simulink subsystem "v2021_10_27_Gear"  (R2020b)
settings: Solver=VariableStepAuto  StartTime=0.0  StopTime=10.0  RelTol=1e-3
values from neighbouring files (symbols this model uses):
  coeffAttritoStatico = 0.7    [v2021_10_27_avvioSITL.m]
  costantiMagicFormula = [ 10 1.3 1 0.95 ]    [v2021_10_27_avvioSITL.m]
  limitAinf = -500    [v2021_10_27_avvioSITL.m]
  limitAup = 500    [v2021_10_27_avvioSITL.m]
  limitPinf = -500    [v2021_10_27_avvioSITL.m]
  limitPup = 500    [v2021_10_27_avvioSITL.m]
  massaRuotaAnteriore = m    [v2021_10_27_avvioSITL.m]
  massaRuotePosteriori = m    [v2021_10_27_avvioSITL.m]
  Zpista = 0    [v2021_10_27_avvioSITL.m]
libraries: sharedutil x12, vrlib x9, simulink x1
(part 1 of 2)
settings Model: Creator=Simone  LastModifiedBy=emanueledalessio

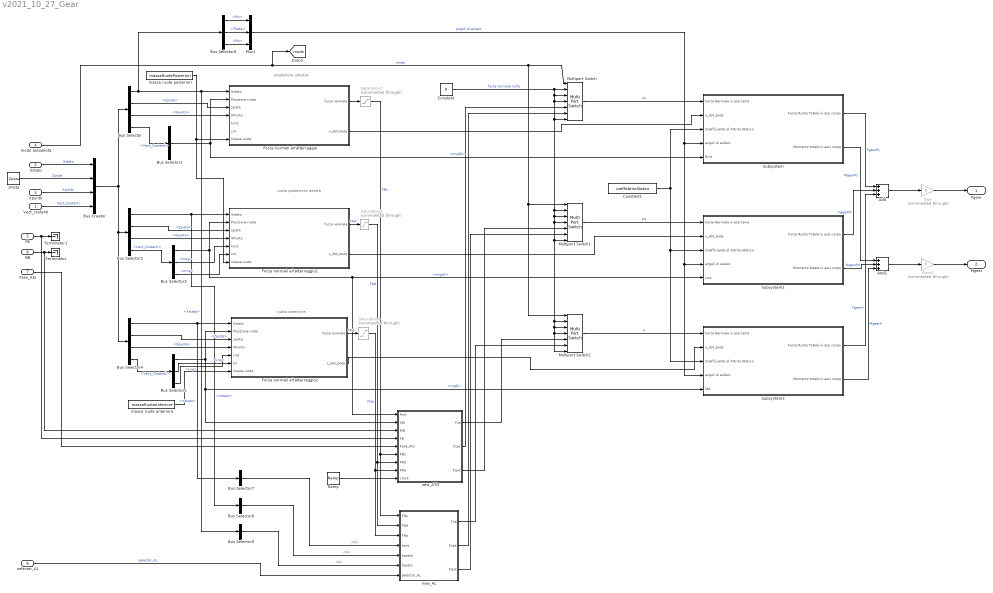
== system v2021_10_27_Gear ==
  note: ruota anteriore
  note: ruota posteriore destra
  note: posteriore sinistra
  Vect_costanti : Inport
  Xstato : Inport  Port=2
  Xpunto : Inport  Port=3
  modo autopilota : Inport  Port=4
  FB : Inport  Port=5
  MB : Inport  Port=6
  Fase_Ato : Inport  Port=7
  selector_AL : Inport  Port=8
  Add : Sum  Inputs=+++
  Add1 : Sum  Inputs=+++
  Bus Creator : BusCreator  Inputs=4
  Bus Selector : BusSelector  OutputSignals=Xstato,Zpista,Xpunto,Vect_Costanti
  Bus Selector1 : BusSelector  OutputSignals=Vett_caratteristici.rmglG
  Bus Selector2 : BusSelector  OutputSignals=Xstato,Zpista,Xpunto,Vect_Costanti
  Bus Selector3 : BusSelector  OutputSignals=Vett_caratteristici.rmgrG,gear.kmg,gear.cmg
  Bus Selector4 : BusSelector  OutputSignals=Xstato,Zpista,Xpunto,Vect_Costanti
  Bus Selector5 : BusSelector  OutputSignals=Vett_caratteristici.rngG,gear.kng,gear.cng
  Bus Selector6 : BusSelector  OutputSignals=PhiThetaPsi.Phi,PhiThetaPsi.Theta,PhiThetaPsi.Psi
  Bus Selector7 : BusSelector  OutputSignals=xyz.h
  Bus Selector8 : BusSelector  OutputSignals=xyz.h
  Bus Selector9 : BusSelector  OutputSignals=xyz.h
  Constant : Constant  Value=0
  Constant1 : Constant  Value=coeffAttritoStatico
  Forze normali all'atterraggio : Subsystem
  Forze normali all'atterraggio1 : Subsystem
  Forze normali all'atterraggio2 : Subsystem
  Gain : Gain  Commented=through  Gain=0
  Gain1 : Gain  Commented=through  Gain=0
  Multiport Switch : MultiPortSwitch  DataPortOrder=Specify indices  DataPortIndices={0,1,2,3,4,5}
  Multiport Switch1 : MultiPortSwitch  DataPortOrder=Specify indices  DataPortIndices={0,1,2,3,4,5}
  Multiport Switch2 : MultiPortSwitch  DataPortOrder=Specify indices  DataPortIndices={0,1,2,3,4,5}
  Mux1 : Mux  Inputs=3
  Ramp : simulink/Sources/Ramp  slope=1  start=0  InitialOutput=0
  Saturation2 : Saturate  Commented=through  UpperLimit=600  LowerLimit=-600
  Saturation3 : Saturate  Commented=through  UpperLimit=600  LowerLimit=-600
  Saturation4 : Saturate  Commented=through  UpperLimit=950  LowerLimit=-950
  Subsystem : Subsystem
  Subsystem1 : Subsystem
  Subsystem2 : Subsystem
  Terminator : Terminator
  Terminator1 : Terminator
  massa ruota anteriore : Constant  Value=massaRuotaAnteriore
  massa ruote posteriori : Constant  Value=massaRuotePosteriori
  new_AL : MATLAB Function  TreatAsAtomicUnit=on
  new_ATO : MATLAB Function  TreatAsAtomicUnit=on
  zPista : Constant  Value=Zpista
  Fgear : Outport  VectorParamsAs1DForOutWhenUnconnected=off
  Mgear : Outport  Port=2  VectorParamsAs1DForOutWhenUnconnected=off
  tag scope: modo=global
  wires:
  Constant1/1 -> Subsystem/3(Coefficiente di Attrito Statico), Subsystem1/3(Coefficiente di Attrito Statico), Subsystem2/3(Coefficiente di Attrito Statico)
  Bus Selector1/1 -> Subsystem/5(Rmt), Forze normali all'atterraggio/2(Posizione ruota)  "<rmglG>"
  Subsystem/2(Momento totale in assi corpo) -> Add1/1  "MgearPs"
  massa ruota anteriore/1 -> Forze normali all'atterraggio2/7(massa ruota)
  Forze normali all'atterraggio/1(forza normale) -> Saturation2/1
  Forze normali all'atterraggio2/2(x_dot_body) -> Subsystem2/2(x_dot_body)
  Forze normali all'atterraggio1/1(forza normale) -> Saturation3/1  "FNd"
  modo autopilota/1 -> Multiport Switch/1, Multiport Switch1/1, Multiport Switch2/1, [modo]  "modo"
  Add/1 -> Gain/1
  Add1/1 -> Gain1/1
  Constant/1 -> Multiport Switch/2, Multiport Switch/3, Multiport Switch1/2, Multiport Switch1/3, Multiport Switch2/2, Multiport Switch2/3, Multiport Switch2/7, Multiport Switch2/4, Multiport Switch1/7, Multiport Switch1/4, Multiport Switch/7, Multiport Switch/4  "forza normale nulla"
  Bus Selector6/2 -> Mux1/2  "<Theta>"
  Bus Selector4/4 -> Bus Selector5/1  "<Vect_Costanti>"
  Subsystem2/2(Momento totale in assi corpo) -> Add1/3  "MgearA"
  ? -> Forze normali all'atterraggio/5(kmd)  "<kmg>"
  Bus Selector5/3 -> Forze normali all'atterraggio2/5(cnd)  "<cng>"
  Bus Selector6/3 -> Mux1/3  "<Psi>"
  Fase_Ato/1 -> new_ATO/5(Fase_Ato)
  Bus Creator/1 -> Bus Selector/1, Bus Selector2/1, Bus Selector4/1
  Bus Selector2/1 -> Forze normali all'atterraggio1/1(Xstato), Bus Selector8/1  "<Xstato>"
  Xpunto/1 -> Bus Creator/3  "Xpunto"
  Bus Selector4/1 -> Forze normali all'atterraggio2/1(Xstato), Bus Selector7/1  "<Xstato>"
  Bus Selector2/4 -> Bus Selector3/1  "<Vect_Costanti>"
  Forze normali all'atterraggio1/2(x_dot_body) -> Subsystem1/2(x_dot_body)
  Xstato/1 -> Bus Creator/1  "Xstato"
  Multiport Switch1/1 -> Subsystem1/1(Forza Normale in assi terra)  "Pd"
  Subsystem1/2(Momento totale in assi corpo) -> Add1/2  "MgearPd"
  Bus Selector/4 -> Bus Selector1/1  "<Vect_Costanti>"
  Multiport Switch/1 -> Subsystem/1(Forza Normale in assi terra)  "Ps"
  Subsystem1/1(Forza Ruota Totale in assi corpo) -> Add/2  "FgearPd"
  Forze normali all'atterraggio/2(x_dot_body) -> Subsystem/2(x_dot_body)
  Subsystem2/1(Forza Ruota Totale in assi corpo) -> Add/3  "FgearA"
  zPista/1 -> Bus Creator/2  "Zpista"
  Bus Selector/1 -> Forze normali all'atterraggio/1(Xstato), Bus Selector9/1, Bus Selector6/1  "<Xstato>"
  massa ruote posteriori/1 -> Forze normali all'atterraggio/7(massa ruota), Forze normali all'atterraggio1/7(massa ruota)
  Bus Selector2/3 -> Forze normali all'atterraggio1/4(XPunto)  "<Xpunto>"
  Bus Selector6/1 -> Mux1/1  "<Phi>"
  ? -> Forze normali all'atterraggio/6(cm)  "<cmg>"
  Bus Selector/3 -> Forze normali all'atterraggio/4(XPunto)  "<Xpunto>"
  Bus Selector5/2 -> Forze normali all'atterraggio2/6(kn)  "<kng>"
  Bus Selector2/2 -> Forze normali all'atterraggio1/3(zpista)  "<Zpista>"
  Bus Selector/2 -> Forze normali all'atterraggio/3(zpista)  "<Zpista>"
  Bus Selector3/1 -> Forze normali all'atterraggio1/2(Posizione ruota), Subsystem1/5(Lmt), new_ATO/1(Rmt)  "<rmgrG>"
  Vect_costanti/1 -> Bus Creator/4  "Vect_Costanti"
  Forze normali all'atterraggio2/1(forza normale) -> Saturation4/1  "FNa"
  Multiport Switch2/1 -> Subsystem2/1(Forza Normale in assi terra)  "A"
  Bus Selector5/1 -> Forze normali all'atterraggio2/2(Posizione ruota), new_ATO/2(Sbt), Subsystem2/5(Sbt)  "<rngG>"
  Subsystem/1(Forza Ruota Totale in assi corpo) -> Add/1  "FgearPs"
  Mux1/1 -> Subsystem/4(angoli di eulero), Subsystem1/4(angoli di eulero), Subsystem2/4(angoli di eulero)  "angoli di eulero"
  Bus Selector4/3 -> Forze normali all'atterraggio2/4(XPunto)  "<Xpunto>"
  Bus Selector4/2 -> Forze normali all'atterraggio2/3(zpista)  "<Zpista>"
  new_ATO/1(Fza) -> Multiport Switch2/5
  Bus Selector3/3 -> Forze normali all'atterraggio1/6(cm)  "<cmg>"
  Bus Selector3/2 -> Forze normali all'atterraggio1/5(kmd)  "<kmg>"
  FB/1 -> Terminator1/1, new_ATO/4(FB)
  Saturation2/1 -> new_AL/1(FNs), new_ATO/6(FNs)  "FNs"
  Saturation3/1 -> new_AL/2(FNd), new_ATO/7(FNd)  "FNd"
  Saturation4/1 -> new_ATO/8(FNa), new_AL/3(FNa)  "FNa"
  new_ATO/2(Fzps) -> Multiport Switch/5
  new_ATO/3(Fzpd) -> Multiport Switch1/5
  Ramp/1 -> new_ATO/9(clock)
  MB/1 -> Terminator/1, new_ATO/3(MB)
  Gain1/1 -> Mgear/1
  Gain/1 -> Fgear/1
  new_AL/1(Fza) -> Multiport Switch2/6
  new_AL/3(Fzpd) -> Multiport Switch1/6
  new_AL/2(Fzps) -> Multiport Switch/6
  Bus Selector7/1 -> new_AL/4(hant)  "<h>"
  Bus Selector8/1 -> new_AL/5(hpostd)  "<h>"
  Bus Selector9/1 -> new_AL/6(hposts)  "<h>"
  selector_AL/1 -> new_AL/7(selector_AL)  "selector_AL"

== system v2021_10_27_Gear/Forze normali all'atterraggio ==
  note: ruota posteriore sinistra
  note: CINEMATICA RUOTE
  Xstato : Inport
  Posizione ruota : Inport  Port=2
  zpista : Inport  Port=3
  XPunto : Inport  Port=4
  kmd : Inport  Port=5
  cm : Inport  Port=6
  massa ruota : Inport  Port=7
  Demux : Demux  Outputs=3
  Demux4 : Demux  Outputs=3
  Subsystem5 : Subsystem
  Terminator{,1..3} (4 alike) : Terminator
  cinematica : Subsystem
  forza normale : Outport
  x_dot_body : Outport  Port=2
  wires:
  cm/1 -> Subsystem5/5(km)
  kmd/1 -> Subsystem5/4(cmd)
  massa ruota/1 -> Subsystem5/6(massa ruota)
  Subsystem5/1(forza normale) -> forza normale/1
  XPunto/1 -> cinematica/4(XPunto)
  zpista/1 -> cinematica/3(Zpista)
  Posizione ruota/1 -> cinematica/2(Posisione Ruota)
  Xstato/1 -> cinematica/1(Xstato)
  cinematica/3(accelerazione ruota rispetto al terreno) -> Demux/1  "x_dot_dot"
  cinematica/1(distanza verticale ruota pista) -> Subsystem5/1(h)  "hps"
  cinematica/2(velocità ruota rispetto al terreno) -> Demux4/1  "x_dot"
  Demux/1 -> Terminator1/1  "x_dot_dot"
  Demux4/2 -> Terminator2/1  "y_dot"
  Demux4/1 -> Terminator3/1  "x_dot"
  Demux4/3 -> Subsystem5/2(h_dot)  "h_dot"
  Demux/3 -> Subsystem5/3(h_dot_dot)  "h_dot dot"
  cinematica/4(velocità ruota rispetto al terreno in assi corpo) -> x_dot_body/1  "x_dot_body"
  Demux/2 -> Terminator/1  "y_dot_dot"

== system v2021_10_27_Gear/Forze normali all'atterraggio1 ==
  note: ruota posteriore sinistra
  note: CINEMATICA RUOTE
  Xstato : Inport
  Posizione ruota : Inport  Port=2
  zpista : Inport  Port=3
  XPunto : Inport  Port=4
  kmd : Inport  Port=5
  cm : Inport  Port=6
  massa ruota : Inport  Port=7
  Demux : Demux  Outputs=3
  Demux4 : Demux  Outputs=3
  Subsystem5 : Subsystem
  Terminator{,1..3} (4 alike) : Terminator
  cinematica : Subsystem
  forza normale : Outport
  x_dot_body : Outport  Port=2
  wires:
  cm/1 -> Subsystem5/5(km)
  kmd/1 -> Subsystem5/4(cmd)
  massa ruota/1 -> Subsystem5/6(massa ruota)
  Subsystem5/1(forza normale) -> forza normale/1
  XPunto/1 -> cinematica/4(XPunto)
  zpista/1 -> cinematica/3(Zpista)
  Posizione ruota/1 -> cinematica/2(Posisione Ruota)
  Xstato/1 -> cinematica/1(Xstato)
  cinematica/3(accelerazione ruota rispetto al terreno) -> Demux/1  "x_dot_dot"
  cinematica/1(distanza verticale ruota pista) -> Subsystem5/1(h)  "hpd"
  cinematica/2(velocità ruota rispetto al terreno) -> Demux4/1  "x_dot"
  Demux/1 -> Terminator1/1  "x_dot_dot"
  Demux4/2 -> Terminator2/1  "y_dot"
  Demux4/1 -> Terminator3/1  "x_dot"
  Demux4/3 -> Subsystem5/2(h_dot)  "h_dot"
  Demux/3 -> Subsystem5/3(h_dot_dot)  "h_dot dot"
  cinematica/4(velocità ruota rispetto al terreno in assi corpo) -> x_dot_body/1  "x_dot_body"
  Demux/2 -> Terminator/1  "y_dot_dot"

== system v2021_10_27_Gear/Forze normali all'atterraggio2 ==
  note: ruota posteriore sinistra
  note: CINEMATICA RUOTE
  Xstato : Inport
  Posizione ruota : Inport  Port=2
  zpista : Inport  Port=3
  XPunto : Inport  Port=4
  cnd : Inport  Port=5
  kn : Inport  Port=6
  massa ruota : Inport  Port=7
  Demux : Demux  Outputs=3
  Demux4 : Demux  Outputs=3
  Subsystem5 : Subsystem
  Terminator{,1..3} (4 alike) : Terminator
  cinematica : Subsystem
  forza normale : Outport
  x_dot_body : Outport  Port=2
  wires:
  kn/1 -> Subsystem5/5(kn)
  cnd/1 -> Subsystem5/4(cnd)
  massa ruota/1 -> Subsystem5/6(massa ruota)
  Subsystem5/1(forza normale) -> forza normale/1
  XPunto/1 -> cinematica/4(XPunto)
  zpista/1 -> cinematica/3(Zpista)
  Posizione ruota/1 -> cinematica/2(Posisione Ruota)
  Xstato/1 -> cinematica/1(Xstato)
  cinematica/3(accelerazione ruota rispetto al terreno) -> Demux/1  "x_dot_dot"
  cinematica/1(distanza verticale ruota pista) -> Subsystem5/1(h)  "ha"
  cinematica/2(velocità ruota rispetto al terreno) -> Demux4/1  "x_dot"
  Demux/1 -> Terminator1/1  "x_dot_dot"
  Demux4/2 -> Terminator2/1  "y_dot"
  Demux4/1 -> Terminator3/1  "x_dot"
  Demux4/3 -> Subsystem5/2(h_dot)  "h_dot"
  Demux/3 -> Subsystem5/3(h_dot_dot)  "h_dot dot"
  cinematica/4(velocità ruota rispetto al terreno in assi corpo) -> x_dot_body/1  "x_dot_body"
  Demux/2 -> Terminator/1  "y_dot_dot"

== system v2021_10_27_Gear/Subsystem ==
  note: di solito: B = 10
      | 		C = 1.3
      | 		D = 1
      | 		E = 0.95
  Forza Normale in assi terra : Inport
  x_dot_body : Inport  Port=2
  Coefficiente di Attrito Statico : Inport  Port=3
  angoli di eulero : Inport  Port=4
  Rmt : Inport  Port=5
  Atan : Trigonometry  Operator=atan
  Constant : Constant  Value=0
  Cross Product : vrlib/Utilities/Cross Product
  Demux : Demux  Outputs=3
  Demux1 : Demux
  Demux2 : Demux  Outputs=3
  Divide : Product  Inputs=*/
  Gain : Gain  Commented=through  Gain=-1
  Gain1 : Gain  Gain=-1
  Gain3 : Gain  Gain=-1
  Gain4 : Gain  Commented=through  Gain=0
  MATLAB Function1 : MATLAB Function  TreatAsAtomicUnit=on
  MATLAB Function3 : MATLAB Function  TreatAsAtomicUnit=on
  Mux : Mux  Inputs=3
  Mux1 : Mux  Inputs=3
  Product : Product
  Saturation : Saturate  UpperLimit=0  LowerLimit=-1000000
  Subsystem : Subsystem
  Terminator : Terminator
  Terminator1 : Terminator
  Terminator2 : Terminator
  Vettore Coefficienti Magic Formula : Constant  Value=costantiMagicFormula  VectorParams1D=off
  Forza Ruota Totale in assi corpo : Outport
  Momento totale in assi corpo : Outport  Port=2
  wires:
  Gain1/1 -> Mux/1
  Gain4/1 -> Mux/3
  Gain3/1 -> Mux1/3
  Forza Normale in assi terra/1 -> Product/1, Gain3/1
  Gain/1 -> Saturation/1
  Saturation/1 -> MATLAB Function1/6(Fa)
  MATLAB Function3/1(forza_normale) -> Gain/1
  Mux1/1 -> Subsystem/2(Input1)
  Demux2/3 -> Gain4/1
  Demux2/2 -> Terminator2/1
  Demux2/1 -> Terminator1/1
  Subsystem/1(Output) -> Demux2/1  "forza normale in assi corpo"
  Product/1 -> MATLAB Function3/1(forzanormale)  "Fa max"
  Demux1/4 -> MATLAB Function1/4(E)  "E"
  Demux1/3 -> MATLAB Function1/3(D)  "D"
  Demux1/2 -> MATLAB Function1/2(C)  "C"
  Demux1/1 -> MATLAB Function1/1(B)  "B"
  Vettore Coefficienti Magic Formula/1 -> Demux1/1
  Cross Product/1 -> Momento totale in assi corpo/1
  Rmt/1 -> Cross Product/1
  angoli di eulero/1 -> Subsystem/1(Input)
  Constant/1 -> Mux1/1, Mux1/2
  Mux/1 -> Forza Ruota Totale in assi corpo/1, Cross Product/2
  MATLAB Function1/2(Fy) -> Mux/2  "Fy"
  MATLAB Function1/1(Fx) -> Gain1/1  "Fx"
  Demux/1 -> Divide/2
  Atan/1 -> MATLAB Function1/5(beta)  "Angolo di Deriva beta"
  Divide/1 -> Atan/1
  Demux/2 -> Divide/1
  Demux/3 -> Terminator/1
  Coefficiente di Attrito Statico/1 -> Product/2
  x_dot_body/1 -> Demux/1  "vettore velocità ruota in assi corpo"

== system v2021_10_27_Gear/Subsystem1 ==
  note: di solito: B = 10
      | 		C = 1.3
      | 		D = 1
      | 		E = 0.95
  Forza Normale in assi terra : Inport
  x_dot_body : Inport  Port=2
  Coefficiente di Attrito Statico : Inport  Port=3
  angoli di eulero : Inport  Port=4
  Lmt : Inport  Port=5
  Atan : Trigonometry  Operator=atan
  Constant : Constant  Value=0
  Cross Product : vrlib/Utilities/Cross Product
  Demux : Demux  Outputs=3
  Demux1 : Demux
  Demux2 : Demux  Outputs=3
  Divide : Product  Inputs=*/
  Gain : Gain  Commented=through  Gain=-1
  Gain1 : Gain  Gain=-1
  Gain3 : Gain  Gain=-1
  Gain4 : Gain  Commented=through  Gain=0
  MATLAB Function1 : MATLAB Function  TreatAsAtomicUnit=on
  MATLAB Function3 : MATLAB Function  TreatAsAtomicUnit=on
  Mux : Mux  Inputs=3
  Mux1 : Mux  Inputs=3
  Product : Product
  Saturation : Saturate  UpperLimit=0  LowerLimit=-1000000
  Subsystem : Subsystem
  Terminator : Terminator
  Terminator1 : Terminator
  Terminator2 : Terminator
  Vettore Coefficienti Magic Formula1 : Constant  Value=costantiMagicFormula  VectorParams1D=off
  Forza Ruota Totale in assi corpo : Outport
  Momento totale in assi corpo : Outport  Port=2
  wires:
  Gain4/1 -> Mux/3
  Gain1/1 -> Mux1/3
  Gain3/1 -> Mux/1
  MATLAB Function3/1(forza_normale) -> Gain/1
  Gain/1 -> Saturation/1
  Saturation/1 -> MATLAB Function1/6(Fa)
  Demux2/3 -> Gain4/1
  Subsystem/1(Output) -> Demux2/1  "forza normale in assi corpo"
  Demux2/2 -> Terminator2/1
  Demux2/1 -> Terminator1/1
  Forza Normale in assi terra/1 -> Gain1/1, Product/1
  Product/1 -> MATLAB Function3/1(forzanormale)  "Fa max"
  Demux1/4 -> MATLAB Function1/4(E)  "E"
  Demux1/3 -> MATLAB Function1/3(D)  "D"
  Demux1/2 -> MATLAB Function1/2(C)  "C"
  Demux1/1 -> MATLAB Function1/1(B)  "B"
  Vettore Coefficienti Magic Formula1/1 -> Demux1/1
  Cross Product/1 -> Momento totale in assi corpo/1
  Lmt/1 -> Cross Product/1
  Mux1/1 -> Subsystem/2(Input1)
  angoli di eulero/1 -> Subsystem/1(Input)
  Constant/1 -> Mux1/1, Mux1/2
  Mux/1 -> Forza Ruota Totale in assi corpo/1, Cross Product/2
  MATLAB Function1/2(Fy) -> Mux/2  "Fy"
  MATLAB Function1/1(Fx) -> Gain3/1  "Fx"
  Demux/1 -> Divide/2
  Atan/1 -> MATLAB Function1/5(beta)  "Angolo di Deriva beta"
  Divide/1 -> Atan/1
  Demux/2 -> Divide/1
  Demux/3 -> Terminator/1
  Coefficiente di Attrito Statico/1 -> Product/2
  x_dot_body/1 -> Demux/1  "vettore velocità ruota in assi corpo"

== system v2021_10_27_Gear/Subsystem2 ==
  note: di solito: B = 10
      | 		C = 1.3
      | 		D = 1
      | 		E = 0.95
  Forza Normale in assi terra : Inport
  x_dot_body : Inport  Port=2
  Coefficiente di Attrito Statico : Inport  Port=3
  angoli di eulero : Inport  Port=4
  Sbt : Inport  Port=5
  Atan : Trigonometry  Operator=atan
  Constant : Constant  Value=0
  Cross Product : vrlib/Utilities/Cross Product
  Demux : Demux  Outputs=3
  Demux1 : Demux
  Demux2 : Demux  Outputs=3
  Divide : Product  Inputs=*/
  Gain : Gain  Commented=through  Gain=-1
  Gain2 : Gain  Gain=-1
  Gain3 : Gain  Gain=-1
  Gain4 : Gain  Commented=through  Gain=0
  MATLAB Function1 : MATLAB Function  TreatAsAtomicUnit=on
  MATLAB Function3 : MATLAB Function  TreatAsAtomicUnit=on
  Mux : Mux  Inputs=3
  Mux1 : Mux  Inputs=3
  Product : Product
  Saturation : Saturate  UpperLimit=0  LowerLimit=-1000000
  Subsystem : Subsystem
  Terminator : Terminator
  Terminator1 : Terminator
  Terminator2 : Terminator
  Vettore Coefficienti Magic Formula : Constant  Value=costantiMagicFormula  VectorParams1D=off
  Forza Ruota Totale in assi corpo : Outport
  Momento totale in assi corpo : Outport  Port=2
  wires:
  Gain4/1 -> Mux/3
  Gain3/1 -> Mux1/3
  Gain2/1 -> Mux/1
  Gain/1 -> Saturation/1
  Saturation/1 -> MATLAB Function1/6(Fa)
  MATLAB Function3/1(forza_normale) -> Gain/1
  Mux1/1 -> Subsystem/2(Input1)
  Demux2/3 -> Gain4/1
  Subsystem/1(Output) -> Demux2/1  "forza normale in assi corpo"
  Demux2/2 -> Terminator2/1
  Demux2/1 -> Terminator1/1
  Forza Normale in assi terra/1 -> Gain3/1, Product/1
  Product/1 -> MATLAB Function3/1(forzanormale)  "Fa max"
  Demux1/4 -> MATLAB Function1/4(E)  "E"
  Demux1/3 -> MATLAB Function1/3(D)  "D"
  Demux1/2 -> MATLAB Function1/2(C)  "C"
  Demux1/1 -> MATLAB Function1/1(B)  "B"
  Vettore Coefficienti Magic Formula/1 -> Demux1/1
  Cross Product/1 -> Momento totale in assi corpo/1
  Sbt/1 -> Cross Product/1
  angoli di eulero/1 -> Subsystem/1(Input)
  Constant/1 -> Mux1/1, Mux1/2
  Mux/1 -> Forza Ruota Totale in assi corpo/1, Cross Product/2
  MATLAB Function1/2(Fy) -> Mux/2  "Fy"
  MATLAB Function1/1(Fx) -> Gain2/1  "Fx"
  Demux/1 -> Divide/2
  Atan/1 -> MATLAB Function1/5(beta)  "Angolo di Deriva beta"
  Divide/1 -> Atan/1
  Demux/2 -> Divide/1
  Demux/3 -> Terminator/1
  Coefficiente di Attrito Statico/1 -> Product/2
  x_dot_body/1 -> Demux/1  "vettore velocità ruota in assi corpo"

== system v2021_10_27_Gear/Forze normali all'atterraggio/Subsystem5 ==
  note: allungamento massimo e minimo ruote posteriori
  note: da mettere a punto anche con l'accelerazione verticale in arrivo dal ciclo, in quanto altrimenti al momento del reset arrivano dati incongruenti uno con l'altro.
  note: Questa era la prima logica di reset sviluppata, da provare.
  h : Inport
  h_dot : Inport  Port=2
  h_dot_dot : Inport  Port=3
  cmd : Inport  Port=4
  km : Inport  Port=5
  massa ruota : Inport  Port=6
  Constant : Constant  Value=10^7
  Constant1 : Constant  Value=0.015
  Constant2 : Constant  Value=0
  Constant3 : Constant  Value=0.89
  Constant4 : Constant  Value=0.12
  Constant5 : Constant  Value=0.3925
  Gain : Gain  Commented=through  Gain=0
  Integrator : Integrator  ExternalReset=level hold  InitialConditionSource=external
  Integrator1 : Integrator  ExternalReset=level hold  InitialConditionSource=external
  Multiport Switch : MultiPortSwitch  DataPortOrder=Specify indices  Inputs=2  DataPortIndices={0,1,2,3,4,5}
  Multiport Switch1 : MultiPortSwitch  DataPortOrder=Specify indices  Inputs=2  DataPortIndices={0,1,2,3,4,5}
  Product : Product
  Product1 : Product
  Saturation : Saturate  UpperLimit=0.015  LowerLimit=-0.0015
  Saturation1 : Saturate  Commented=through  UpperLimit=0.1  LowerLimit=-0.001
  Saturation2 : Saturate  UpperLimit=limitPup  LowerLimit=limitPinf
  Sum : Sum  Inputs=|+-
  Sum1 : Sum  Inputs=+-
  Sum2 : Sum  Inputs=|++
  Sum3 : Sum
  Sum5 : Sum  Inputs=|++
  divisione per massa ruota : Product  Inputs=*/
  h * km molla : Product
  logica reset : Subsystem  Commented=through
  logica reset1 : Subsystem  Commented=through
  v * cmd smorzamento : Product
  forza normale : Outport
  wires:
  Multiport Switch1/1 -> Sum5/1
  Constant2/1 -> Multiport Switch1/3, Multiport Switch1/4, Multiport Switch1/2, Multiport Switch1/5, Multiport Switch1/7
  Constant5/1 -> Multiport Switch1/6
  [modo] -> Multiport Switch1/1
  h/1 -> Sum5/2  "h"
  Sum5/1 -> Integrator1/3, logica reset/1(Input)
  Product1/1 -> divisione per massa ruota/1, forza normale/1
  Saturation2/1 -> Product1/1
  Constant4/1 -> Multiport Switch/5
  Multiport Switch/1 -> Product1/2
  Constant3/1 -> Multiport Switch/2, Multiport Switch/3, Multiport Switch/4, Multiport Switch/6, Multiport Switch/7
  [modo] -> Multiport Switch/1
  Sum2/1 -> Sum3/2  "forza molla"
  logica reset/1(Output) -> Gain/1, Integrator1/2  "segnale di reset"
  Gain/1 -> Integrator/2
  cmd/1 -> v * cmd smorzamento/2
  h * km molla/1 -> Sum2/2
  Product/1 -> Sum2/1
  Constant/1 -> Product/2
  Saturation1/1 -> Product/1
  Sum/1 -> Saturation1/1
  Constant1/1 -> Sum/2
  Saturation/1 -> h * km molla/1
  massa ruota/1 -> divisione per massa ruota/2
  h_dot/1 -> Integrator/3  "h_dot"
  km/1 -> h * km molla/2
  Sum3/1 -> Saturation2/1  "forze"
  v * cmd smorzamento/1 -> Sum3/1  "forza smorzatore"
  Integrator1/1 -> Saturation/1, Sum/1  "h"
  h_dot_dot/1 -> Sum1/1  "h_dot_dot"
  divisione per massa ruota/1 -> Sum1/2
  Sum1/1 -> Integrator/1  "h_dot_dot"
  Integrator/1 -> v * cmd smorzamento/1, Integrator1/1  "h_dot"

== system v2021_10_27_Gear/Forze normali all'atterraggio/cinematica ==
  note: velocità Cg in assi corpo
  Xstato : Inport
  Posisione Ruota : Inport  Port=2
  Zpista : Inport  Port=3
  XPunto : Inport  Port=4
  Bus Selector : BusSelector  OutputSignals=Vbpunto,ωpunto
  Bus Selector1 : BusSelector  OutputSignals=xyz.x,xyz.y,xyz.h
  Bus Selector3 : BusSelector  OutputSignals=ωvect
  Bus Selector6 : BusSelector  OutputSignals=PhiThetaPsi.Phi,PhiThetaPsi.Theta,PhiThetaPsi.Psi
  Bus Selector7 : BusSelector  OutputSignals=uvw
  Cross Product1 : vrlib/Utilities/Cross Product
  Cross Product2 : vrlib/Utilities/Cross Product
  Demux : Demux  Outputs=3
  Demux1 : Demux  Outputs=3
  Mux : Mux  Inputs=3
  Mux1 : Mux  Inputs=3
  Subsystem : Subsystem
  Subsystem1 : Subsystem
  Subsystem2 : Subsystem
  Sum : Sum  Inputs=|-++
  Sum1 : Sum  Inputs=|++
  Sum2 : Sum  Inputs=|++
  Terminator{,1,4..5} (4 alike) : Terminator
  distanza verticale ruota pista : Outport
  velocità ruota rispetto al terreno : Outport  Port=2
  accelerazione ruota rispetto al terreno : Outport  Port=3
  velocità ruota rispetto al terreno in assi corpo : Outport  Port=4
  wires:
  Subsystem2/1(Output) -> accelerazione ruota rispetto al terreno/1  "accelerazione ruota rispetto al terreno in assi terra"
  Sum/1 -> distanza verticale ruota pista/1  "altezza ruota pista"
  Demux1/3 -> Sum/2  "z ruota rispetto al Cg in assi terra"
  Demux1/2 -> Terminator1/1
  Demux1/1 -> Terminator/1
  Subsystem/1(Output) -> Demux1/1  "posizione ruota rispetto al Cg in assi terra"
  Subsystem1/1(Output) -> velocità ruota rispetto al terreno/1  "velocità ruota rispetto al terreno in assi terra"
  Mux/1 -> Subsystem/2(Input1), Cross Product1/1, Cross Product2/1
  Bus Selector1/3 -> Sum/3  "<h>"
  Bus Selector1/1 -> Terminator5/1  "<x>"
  Demux/3 -> Mux/3  "zps"
  Xstato/1 -> Bus Selector7/1, Bus Selector3/1, Bus Selector6/1, Bus Selector1/1
  Demux/2 -> Mux/2  "yps"
  Bus Selector6/2 -> Mux1/2  "<Theta>"
  Sum1/1 -> velocità ruota rispetto al terreno in assi corpo/1, Subsystem1/2(Input1)  "velocità ruota rispetto al terreno in assi corpo"
  Bus Selector3/1 -> Cross Product1/2  "<ωvect>"
  Posisione Ruota/1 -> Demux/1
  Demux/1 -> Mux/1  "xps"
  Bus Selector6/1 -> Mux1/1  "<Phi>"
  Bus Selector1/2 -> Terminator4/1  "<y>"
  Zpista/1 -> Sum/1
  Bus Selector7/1 -> Sum1/2  "<uvw>"
  Mux1/1 -> Subsystem1/1(Input), Subsystem2/1(Input), Subsystem/1(Input)  "angoli di eulero"
  XPunto/1 -> Bus Selector/1  "accelerazioni"
  Cross Product1/1 -> Sum1/1  "velocità ruota rispetto al baricentro in assi corpo"
  Bus Selector/1 -> Sum2/1  "<Vbpunto>"
  Bus Selector6/3 -> Mux1/3  "<Psi>"
  Sum2/1 -> Subsystem2/2(Input1)  "accelerazione ruota rispetto al terreno in assi corpo"
  Bus Selector/2 -> Cross Product2/2  "<ωpunto>"
  Cross Product2/1 -> Sum2/2

== system v2021_10_27_Gear/Forze normali all'atterraggio1/Subsystem5 ==
  note: allungamento massimo e minimo ruote posteriori
  h : Inport
  h_dot : Inport  Port=2
  h_dot_dot : Inport  Port=3
  cmd : Inport  Port=4
  km : Inport  Port=5
  massa ruota : Inport  Port=6
  Constant : Constant  Value=10^7
  Constant1 : Constant  Value=0.015
  Constant2 : Constant  Value=0
  Constant3 : Constant  Value=0.89
  Constant4 : Constant  Value=0.12
  Constant5 : Constant  Value=0.3925
  Gain : Gain  Commented=through  Gain=0
  Integrator : Integrator  ExternalReset=level hold  InitialConditionSource=external
  Integrator1 : Integrator  ExternalReset=level hold  InitialConditionSource=external
  Multiport Switch : MultiPortSwitch  DataPortOrder=Specify indices  Inputs=2  DataPortIndices={0,1,2,3,4,5}
  Multiport Switch1 : MultiPortSwitch  DataPortOrder=Specify indices  Inputs=2  DataPortIndices={0,1,2,3,4,5}
  Product : Product
  Product1 : Product
  Saturation : Saturate  UpperLimit=0.015  LowerLimit=-0.0015
  Saturation1 : Saturate  Commented=through  UpperLimit=0.1  LowerLimit=-0.001
  Saturation2 : Saturate  UpperLimit=limitPup  LowerLimit=limitPinf
  Sum : Sum  Inputs=|+-
  Sum1 : Sum  Inputs=+-
  Sum2 : Sum  Inputs=|++
  Sum3 : Sum
  Sum5 : Sum  Inputs=|++
  divisione per massa ruota : Product  Inputs=*/
  h * km molla : Product
  logica reset : Subsystem  Commented=through
  v * cmd smorzamento : Product
  forza normale : Outport
  wires:
  Constant2/1 -> Multiport Switch1/3, Multiport Switch1/4, Multiport Switch1/2, Multiport Switch1/5, Multiport Switch1/7
  Constant5/1 -> Multiport Switch1/6
  Multiport Switch1/1 -> Sum5/1
  [modo] -> Multiport Switch1/1
  h/1 -> Sum5/2  "h"
  Sum5/1 -> Integrator1/3, logica reset/1(Input)
  Product1/1 -> divisione per massa ruota/1, forza normale/1
  Saturation2/1 -> Product1/1
  Constant4/1 -> Multiport Switch/5
  [modo] -> Multiport Switch/1
  Constant3/1 -> Multiport Switch/2, Multiport Switch/3, Multiport Switch/4, Multiport Switch/6, Multiport Switch/7
  Multiport Switch/1 -> Product1/2
  Sum2/1 -> Sum3/2
  logica reset/1(Output) -> Gain/1, Integrator1/2  "segnale di reset"
  Gain/1 -> Integrator/2
  h * km molla/1 -> Sum2/2
  Saturation1/1 -> Product/1
  Integrator1/1 -> Saturation/1, Sum/1  "h"
  Product/1 -> Sum2/1
  Sum/1 -> Saturation1/1
  Constant1/1 -> Sum/2
  Constant/1 -> Product/2
  Saturation/1 -> h * km molla/1
  massa ruota/1 -> divisione per massa ruota/2
  km/1 -> h * km molla/2
  Sum3/1 -> Saturation2/1  "forze"
  v * cmd smorzamento/1 -> Sum3/1  "forza smorzatore"
  h_dot_dot/1 -> Sum1/1  "h_dot_dot"
  divisione per massa ruota/1 -> Sum1/2
  Sum1/1 -> Integrator/1  "h_dot_dot"
  Integrator/1 -> v * cmd smorzamento/1, Integrator1/1  "h_dot"
  cmd/1 -> v * cmd smorzamento/2
  h_dot/1 -> Integrator/3  "h_dot"

== system v2021_10_27_Gear/Forze normali all'atterraggio1/cinematica ==
  note: velocità Cg in assi corpo
  Xstato : Inport
  Posisione Ruota : Inport  Port=2
  Zpista : Inport  Port=3
  XPunto : Inport  Port=4
  Bus Selector : BusSelector  OutputSignals=Vbpunto,ωpunto
  Bus Selector1 : BusSelector  OutputSignals=xyz.x,xyz.y,xyz.h
  Bus Selector3 : BusSelector  OutputSignals=ωvect
  Bus Selector6 : BusSelector  OutputSignals=PhiThetaPsi.Phi,PhiThetaPsi.Theta,PhiThetaPsi.Psi
  Bus Selector7 : BusSelector  OutputSignals=uvw
  Cross Product1 : vrlib/Utilities/Cross Product
  Cross Product2 : vrlib/Utilities/Cross Product
  Demux : Demux  Outputs=3
  Demux1 : Demux  Outputs=3
  Mux : Mux  Inputs=3
  Mux1 : Mux  Inputs=3
  Subsystem : Subsystem
  Subsystem1 : Subsystem
  Subsystem2 : Subsystem
  Sum : Sum  Inputs=|-++
  Sum1 : Sum  Inputs=|++
  Sum2 : Sum  Inputs=|++
  Terminator{,1,4..5} (4 alike) : Terminator
  distanza verticale ruota pista : Outport
  velocità ruota rispetto al terreno : Outport  Port=2
  accelerazione ruota rispetto al terreno : Outport  Port=3
  velocità ruota rispetto al terreno in assi corpo : Outport  Port=4
  wires:
  Subsystem2/1(Output) -> accelerazione ruota rispetto al terreno/1  "accelerazione ruota rispetto al terreno in assi terra"
  Sum/1 -> distanza verticale ruota pista/1  "altezza ruota pista"
  Demux1/3 -> Sum/2  "z ruota rispetto al Cg in assi terra"
  Demux1/2 -> Terminator1/1
  Demux1/1 -> Terminator/1
  Subsystem/1(Output) -> Demux1/1  "posizione ruota rispetto al Cg in assi terra"
  Subsystem1/1(Output) -> velocità ruota rispetto al terreno/1  "velocità ruota rispetto al terreno in assi terra"
  Mux/1 -> Cross Product1/1, Cross Product2/1, Subsystem/2(Input1)
  Bus Selector1/3 -> Sum/3  "<h>"
  Bus Selector1/1 -> Terminator5/1  "<x>"
  Demux/3 -> Mux/3  "zps"
  Xstato/1 -> Bus Selector7/1, Bus Selector3/1, Bus Selector6/1, Bus Selector1/1
  Demux/2 -> Mux/2  "yps"
  Bus Selector6/2 -> Mux1/2  "<Theta>"
  Sum1/1 -> velocità ruota rispetto al terreno in assi corpo/1, Subsystem1/2(Input1)  "velocità ruota rispetto al terreno in assi corpo"
  Bus Selector3/1 -> Cross Product1/2  "<ωvect>"
  Posisione Ruota/1 -> Demux/1
  Demux/1 -> Mux/1  "xps"
  Bus Selector6/1 -> Mux1/1  "<Phi>"
  Bus Selector1/2 -> Terminator4/1  "<y>"
  Zpista/1 -> Sum/1
  Bus Selector7/1 -> Sum1/2  "<uvw>"
  Mux1/1 -> Subsystem1/1(Input), Subsystem2/1(Input), Subsystem/1(Input)  "angoli di eulero"
  XPunto/1 -> Bus Selector/1  "accelerazioni"
  Cross Product1/1 -> Sum1/1  "velocità ruota rispetto al baricentro in assi corpo"
  Bus Selector/1 -> Sum2/1  "<Vbpunto>"
  Bus Selector6/3 -> Mux1/3  "<Psi>"
  Sum2/1 -> Subsystem2/2(Input1)  "accelerazione ruota rispetto al terreno in assi corpo"
  Bus Selector/2 -> Cross Product2/2  "<ωpunto>"
  Cross Product2/1 -> Sum2/2

== system v2021_10_27_Gear/Forze normali all'atterraggio2/Subsystem5 ==
  note: allungamento massimo e minimo ruota anteriore
  h : Inport
  h_dot : Inport  Port=2
  h_dot_dot : Inport  Port=3
  cnd : Inport  Port=4
  kn : Inport  Port=5
  massa ruota : Inport  Port=6
  Constant : Constant  Value=8.75*10^3
  Constant1 : Constant  Value=0.03
  Constant2 : Constant  Value=0
  Constant3 : Constant  Value=0.89
  Constant4 : Constant  Value=0.12
  Constant5 : Constant  Value=0.3925
  Gain : Gain  Commented=through  Gain=0
  Integrator : Integrator  ExternalReset=level hold  InitialConditionSource=external
  Integrator1 : Integrator  ExternalReset=level hold  InitialConditionSource=external
  Multiport Switch : MultiPortSwitch  DataPortOrder=Specify indices  Inputs=2  DataPortIndices={0,1,2,3,4,5}
  Multiport Switch1 : MultiPortSwitch  DataPortOrder=Specify indices  Inputs=2  DataPortIndices={0,1,2,3,4,5}
  Product : Product
  Product1 : Product
  Saturation : Saturate  UpperLimit=0.03  LowerLimit=-0.003
  Saturation1 : Saturate  Commented=through  UpperLimit=0.1  LowerLimit=-0.0005
  Saturation2 : Saturate  UpperLimit=limitAup  LowerLimit=limitAinf
  Sum : Sum  Inputs=|+-
  Sum1 : Sum  Inputs=+-
  Sum2 : Sum  Inputs=|++
  Sum3 : Sum
  Sum4 : Sum  Inputs=|++
  divisione per massa ruota : Product  Inputs=*/
  h * kn molla : Product
  logica reset : Subsystem  Commented=through
  v * cnd smorzamento : Product
  forza normale : Outport
  wires:
  Multiport Switch1/1 -> Sum4/1
  Constant2/1 -> Multiport Switch1/3, Multiport Switch1/4, Multiport Switch1/2, Multiport Switch1/5, Multiport Switch1/7
  Constant5/1 -> Multiport Switch1/6
  [modo] -> Multiport Switch1/1
  Sum4/1 -> Integrator1/3, logica reset/1(Input)
  Constant4/1 -> Multiport Switch/5
  [modo] -> Multiport Switch/1
  Product1/1 -> divisione per massa ruota/1, forza normale/1
  Constant3/1 -> Multiport Switch/7, Multiport Switch/2, Multiport Switch/3, Multiport Switch/4, Multiport Switch/6
  Multiport Switch/1 -> Product1/2
  Sum2/1 -> Sum3/2
  logica reset/1(Output) -> Gain/1, Integrator1/2  "segnale di reset"
  Gain/1 -> Integrator/2
  Saturation2/1 -> Product1/1
  cnd/1 -> v * cnd smorzamento/2
  h * kn molla/1 -> Sum2/2
  Saturation1/1 -> Product/1
  Integrator1/1 -> Saturation/1, Sum/1  "h"
  Product/1 -> Sum2/1
  Sum/1 -> Saturation1/1
  Constant1/1 -> Sum/2
  Constant/1 -> Product/2
  Saturation/1 -> h * kn molla/1
  massa ruota/1 -> divisione per massa ruota/2
  h_dot/1 -> Integrator/3  "h_dot"
  kn/1 -> h * kn molla/2
  Sum3/1 -> Saturation2/1  "forze"
  v * cnd smorzamento/1 -> Sum3/1  "forza smorzatore"
  h_dot_dot/1 -> Sum1/1  "h_dot_dot"
  divisione per massa ruota/1 -> Sum1/2
  Sum1/1 -> Integrator/1  "h_dot_dot"
  Integrator/1 -> v * cnd smorzamento/1, Integrator1/1  "h_dot"
  h/1 -> Sum4/2  "h"

== system v2021_10_27_Gear/Forze normali all'atterraggio2/cinematica ==
  note: velocità Cg in assi corpo
  Xstato : Inport
  Posisione Ruota : Inport  Port=2
  Zpista : Inport  Port=3
  XPunto : Inport  Port=4
  Bus Selector : BusSelector  OutputSignals=Vbpunto,ωpunto
  Bus Selector1 : BusSelector  OutputSignals=xyz.x,xyz.y,xyz.h
  Bus Selector3 : BusSelector  OutputSignals=ωvect
  Bus Selector6 : BusSelector  OutputSignals=PhiThetaPsi.Phi,PhiThetaPsi.Theta,PhiThetaPsi.Psi
  Bus Selector7 : BusSelector  OutputSignals=uvw
  Cross Product1 : vrlib/Utilities/Cross Product
  Cross Product2 : vrlib/Utilities/Cross Product
  Demux : Demux  Outputs=3
  Demux1 : Demux  Outputs=3
  Mux : Mux  Inputs=3
  Mux1 : Mux  Inputs=3
  Subsystem : Subsystem
  Subsystem1 : Subsystem
  Subsystem2 : Subsystem
  Sum : Sum  Inputs=|-++
  Sum1 : Sum  Inputs=|++
  Sum2 : Sum  Inputs=|++
  Terminator{,1,4..5} (4 alike) : Terminator
  distanza verticale ruota pista : Outport
  velocità ruota rispetto al terreno : Outport  Port=2
  accelerazione ruota rispetto al terreno : Outport  Port=3
  velocità ruota rispetto al terreno in assi corpo : Outport  Port=4
  wires:
  Subsystem2/1(Output) -> accelerazione ruota rispetto al terreno/1  "accelerazione ruota rispetto al terreno in assi terra"
  Sum/1 -> distanza verticale ruota pista/1  "altezza ruota pista"
  Demux1/3 -> Sum/2  "z ruota rispetto al Cg in assi terra"
  Demux1/2 -> Terminator1/1
  Demux1/1 -> Terminator/1
  Subsystem/1(Output) -> Demux1/1  "posizione ruota rispetto al Cg in assi terra"
  Subsystem1/1(Output) -> velocità ruota rispetto al terreno/1  "velocità ruota rispetto al terreno in assi terra"
  Mux/1 -> Cross Product1/1, Cross Product2/1, Subsystem/2(Input1)
  Bus Selector1/3 -> Sum/3  "<h>"
  Bus Selector1/1 -> Terminator5/1  "<x>"
  Demux/3 -> Mux/3  "zps"
  Xstato/1 -> Bus Selector7/1, Bus Selector3/1, Bus Selector6/1, Bus Selector1/1
  Demux/2 -> Mux/2  "yps"
  Bus Selector6/2 -> Mux1/2  "<Theta>"
  Sum1/1 -> velocità ruota rispetto al terreno in assi corpo/1, Subsystem1/2(Input1)  "velocità ruota rispetto al terreno in assi corpo"
  Bus Selector3/1 -> Cross Product1/2  "<ωvect>"
  Posisione Ruota/1 -> Demux/1
  Demux/1 -> Mux/1  "xps"
  Bus Selector6/1 -> Mux1/1  "<Phi>"
  Bus Selector1/2 -> Terminator4/1  "<y>"
  Zpista/1 -> Sum/1
  Bus Selector7/1 -> Sum1/2  "<uvw>"
  Mux1/1 -> Subsystem1/1(Input), Subsystem2/1(Input), Subsystem/1(Input)  "angoli di eulero"
  XPunto/1 -> Bus Selector/1  "accelerazioni"
  Cross Product1/1 -> Sum1/1  "velocità ruota rispetto al baricentro in assi corpo"
  Bus Selector/1 -> Sum2/1  "<Vbpunto>"
  Bus Selector6/3 -> Mux1/3  "<Psi>"
  Sum2/1 -> Subsystem2/2(Input1)  "accelerazione ruota rispetto al terreno in assi corpo"
  Bus Selector/2 -> Cross Product2/2  "<ωpunto>"
  Cross Product2/1 -> Sum2/2

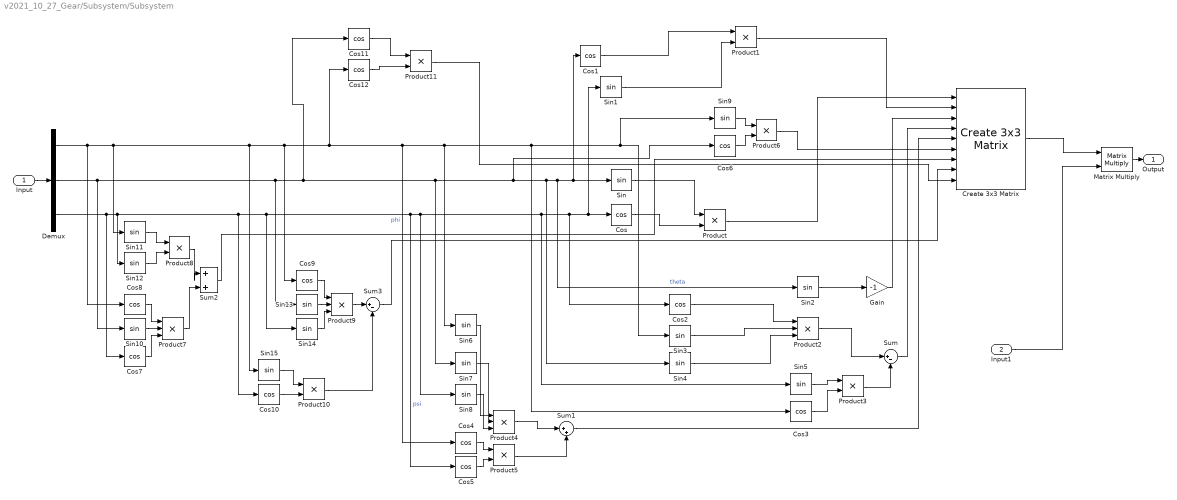
== system v2021_10_27_Gear/Subsystem/Subsystem ==
  Input : Inport
  Input1 : Inport  Port=2
  Cos{,1..12} (13 alike) : Trigonometry  Operator=cos
  Create 3x3 Matrix : sharedutil/Create 3x3 Matrix  aMode=aMode
  Demux : Demux  Outputs=3
  Gain : Gain  Gain=-1
  Matrix Multiply : Product  Multiplication=Matrix(*)
  Product{,1,3,5..6,8,10..11} (8 alike) : Product
  Product{2,4,7,9} (4 alike) : Product  Inputs=3
  Sin{,1..15} (16 alike) : Trigonometry
  Sum : Sum  Inputs=|+-
  Sum1 : Sum  Inputs=|++
  Sum2 : Sum  Inputs=|++
  Sum3 : Sum  Inputs=|+-
  Output : Outport  VectorParamsAs1DForOutWhenUnconnected=off
  wires:
  Matrix Multiply/1 -> Output/1
  Input1/1 -> Matrix Multiply/2
  Create 3x3 Matrix/1 -> Matrix Multiply/1
  Product11/1 -> Create 3x3 Matrix/9
  Cos12/1 -> Product11/2
  Cos11/1 -> Product11/1
  Sum3/1 -> Create 3x3 Matrix/8
  Product10/1 -> Sum3/2
  Cos10/1 -> Product10/2
  Sin15/1 -> Product10/1
  Product9/1 -> Sum3/1
  Sin14/1 -> Product9/3
  Sin13/1 -> Product9/2
  Cos9/1 -> Product9/1
  Sum2/1 -> Create 3x3 Matrix/7
  Product8/1 -> Sum2/1
  Product7/1 -> Sum2/2
  Sin12/1 -> Product8/2
  Sin11/1 -> Product8/1
  Cos7/1 -> Product7/3
  Sin10/1 -> Product7/2
  Cos8/1 -> Product7/1
  Product6/1 -> Create 3x3 Matrix/6
  Cos6/1 -> Product6/2
  Sin9/1 -> Product6/1
  Sum1/1 -> Create 3x3 Matrix/5
  Product5/1 -> Sum1/2
  Product4/1 -> Sum1/1
  Cos5/1 -> Product5/2
  Cos4/1 -> Product5/1
  Sin8/1 -> Product4/3
  Sin7/1 -> Product4/2
  Sin6/1 -> Product4/1
  Sum/1 -> Create 3x3 Matrix/4
  Product3/1 -> Sum/2
  Cos3/1 -> Product3/2
  Sin5/1 -> Product3/1
  Sin4/1 -> Product2/3
  Cos2/1 -> Product2/1
  Product2/1 -> Sum/1
  Sin3/1 -> Product2/2
  Gain/1 -> Create 3x3 Matrix/3
  Demux/2 -> Sin/1, Cos1/1, Sin2/1, Sin4/1, Cos6/1, Sin7/1, Cos11/1, Sin13/1, Sin10/1  "theta"
  Sin2/1 -> Gain/1
  Product1/1 -> Create 3x3 Matrix/2
  Sin1/1 -> Product1/2
  Cos1/1 -> Product1/1
  Product/1 -> Create 3x3 Matrix/1
  Cos/1 -> Product/2
  Sin/1 -> Product/1
  Demux/3 -> Cos/1, Sin1/1, Cos2/1, Sin5/1, Sin8/1, Cos5/1, Sin14/1, Cos10/1, Sin12/1, Cos7/1  "psi"
  Demux/1 -> Sin11/1, Sin3/1, Sin9/1, Cos3/1, Sin6/1, Cos4/1, Cos12/1, Cos9/1, Sin15/1, Cos8/1  "phi"
  Input/1 -> Demux/1

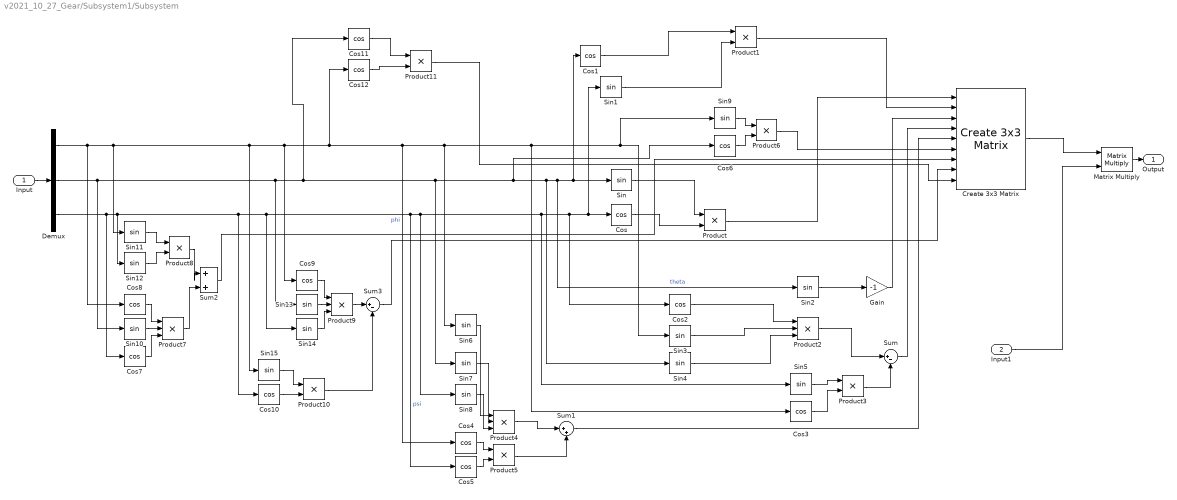
== system v2021_10_27_Gear/Subsystem1/Subsystem ==
  Input : Inport
  Input1 : Inport  Port=2
  Cos{,1..12} (13 alike) : Trigonometry  Operator=cos
  Create 3x3 Matrix : sharedutil/Create 3x3 Matrix  aMode=aMode
  Demux : Demux  Outputs=3
  Gain : Gain  Gain=-1
  Matrix Multiply : Product  Multiplication=Matrix(*)
  Product{,1,3,5..6,8,10..11} (8 alike) : Product
  Product{2,4,7,9} (4 alike) : Product  Inputs=3
  Sin{,1..15} (16 alike) : Trigonometry
  Sum : Sum  Inputs=|+-
  Sum1 : Sum  Inputs=|++
  Sum2 : Sum  Inputs=|++
  Sum3 : Sum  Inputs=|+-
  Output : Outport  VectorParamsAs1DForOutWhenUnconnected=off
  wires:
  Matrix Multiply/1 -> Output/1
  Input1/1 -> Matrix Multiply/2
  Create 3x3 Matrix/1 -> Matrix Multiply/1
  Product11/1 -> Create 3x3 Matrix/9
  Cos12/1 -> Product11/2
  Cos11/1 -> Product11/1
  Sum3/1 -> Create 3x3 Matrix/8
  Product10/1 -> Sum3/2
  Cos10/1 -> Product10/2
  Sin15/1 -> Product10/1
  Product9/1 -> Sum3/1
  Sin14/1 -> Product9/3
  Sin13/1 -> Product9/2
  Cos9/1 -> Product9/1
  Sum2/1 -> Create 3x3 Matrix/7
  Product8/1 -> Sum2/1
  Product7/1 -> Sum2/2
  Sin12/1 -> Product8/2
  Sin11/1 -> Product8/1
  Cos7/1 -> Product7/3
  Sin10/1 -> Product7/2
  Cos8/1 -> Product7/1
  Product6/1 -> Create 3x3 Matrix/6
  Cos6/1 -> Product6/2
  Sin9/1 -> Product6/1
  Sum1/1 -> Create 3x3 Matrix/5
  Product5/1 -> Sum1/2
  Product4/1 -> Sum1/1
  Cos5/1 -> Product5/2
  Cos4/1 -> Product5/1
  Sin8/1 -> Product4/3
  Sin7/1 -> Product4/2
  Sin6/1 -> Product4/1
  Sum/1 -> Create 3x3 Matrix/4
  Product3/1 -> Sum/2
  Cos3/1 -> Product3/2
  Sin5/1 -> Product3/1
  Sin4/1 -> Product2/3
  Cos2/1 -> Product2/1
  Product2/1 -> Sum/1
  Sin3/1 -> Product2/2
  Gain/1 -> Create 3x3 Matrix/3
  Demux/2 -> Sin/1, Cos1/1, Sin2/1, Sin4/1, Cos6/1, Sin7/1, Cos11/1, Sin13/1, Sin10/1  "theta"
  Sin2/1 -> Gain/1
  Product1/1 -> Create 3x3 Matrix/2
  Sin1/1 -> Product1/2
  Cos1/1 -> Product1/1
  Product/1 -> Create 3x3 Matrix/1
  Cos/1 -> Product/2
  Sin/1 -> Product/1
  Demux/3 -> Cos/1, Sin1/1, Cos2/1, Sin5/1, Sin8/1, Cos5/1, Sin14/1, Cos10/1, Sin12/1, Cos7/1  "psi"
  Demux/1 -> Sin11/1, Sin3/1, Sin9/1, Cos3/1, Sin6/1, Cos4/1, Cos12/1, Cos9/1, Sin15/1, Cos8/1  "phi"
  Input/1 -> Demux/1

== system v2021_10_27_Gear/Subsystem2/Subsystem ==
  Input : Inport
  Input1 : Inport  Port=2
  Cos{,1..12} (13 alike) : Trigonometry  Operator=cos
  Create 3x3 Matrix : sharedutil/Create 3x3 Matrix  aMode=aMode
  Demux : Demux  Outputs=3
  Gain : Gain  Gain=-1
  Matrix Multiply : Product  Multiplication=Matrix(*)
  Product{,1,3,5..6,8,10..11} (8 alike) : Product
  Product{2,4,7,9} (4 alike) : Product  Inputs=3
  Sin{,1..15} (16 alike) : Trigonometry
  Sum : Sum  Inputs=|+-
  Sum1 : Sum  Inputs=|++
  Sum2 : Sum  Inputs=|++
  Sum3 : Sum  Inputs=|+-
  Output : Outport  VectorParamsAs1DForOutWhenUnconnected=off
  wires:
  Matrix Multiply/1 -> Output/1
  Input1/1 -> Matrix Multiply/2
  Create 3x3 Matrix/1 -> Matrix Multiply/1
  Product11/1 -> Create 3x3 Matrix/9
  Cos12/1 -> Product11/2
  Cos11/1 -> Product11/1
  Sum3/1 -> Create 3x3 Matrix/8
  Product10/1 -> Sum3/2
  Cos10/1 -> Product10/2
  Sin15/1 -> Product10/1
  Product9/1 -> Sum3/1
  Sin14/1 -> Product9/3
  Sin13/1 -> Product9/2
  Cos9/1 -> Product9/1
  Sum2/1 -> Create 3x3 Matrix/7
  Product8/1 -> Sum2/1
  Product7/1 -> Sum2/2
  Sin12/1 -> Product8/2
  Sin11/1 -> Product8/1
  Cos7/1 -> Product7/3
  Sin10/1 -> Product7/2
  Cos8/1 -> Product7/1
  Product6/1 -> Create 3x3 Matrix/6
  Cos6/1 -> Product6/2
  Sin9/1 -> Product6/1
  Sum1/1 -> Create 3x3 Matrix/5
  Product5/1 -> Sum1/2
  Product4/1 -> Sum1/1
  Cos5/1 -> Product5/2
  Cos4/1 -> Product5/1
  Sin8/1 -> Product4/3
  Sin7/1 -> Product4/2
  Sin6/1 -> Product4/1
  Sum/1 -> Create 3x3 Matrix/4
  Product3/1 -> Sum/2
  Cos3/1 -> Product3/2
  Sin5/1 -> Product3/1
  Sin4/1 -> Product2/3
  Cos2/1 -> Product2/1
  Product2/1 -> Sum/1
  Sin3/1 -> Product2/2
  Gain/1 -> Create 3x3 Matrix/3
  Demux/2 -> Sin/1, Cos1/1, Sin2/1, Sin4/1, Cos6/1, Sin7/1, Cos11/1, Sin13/1, Sin10/1  "theta"
  Sin2/1 -> Gain/1
  Product1/1 -> Create 3x3 Matrix/2
  Sin1/1 -> Product1/2
  Cos1/1 -> Product1/1
  Product/1 -> Create 3x3 Matrix/1
  Cos/1 -> Product/2
  Sin/1 -> Product/1
  Demux/3 -> Cos/1, Sin1/1, Cos2/1, Sin5/1, Sin8/1, Cos5/1, Sin14/1, Cos10/1, Sin12/1, Cos7/1  "psi"
  Demux/1 -> Sin11/1, Sin3/1, Sin9/1, Cos3/1, Sin6/1, Cos4/1, Cos12/1, Cos9/1, Sin15/1, Cos8/1  "phi"
  Input/1 -> Demux/1

== system v2021_10_27_Gear/Forze normali all'atterraggio/Subsystem5/logica reset ==
  Input : Inport
  Constant : Constant  Value=0
  Pulse Generator : DiscretePulseGenerator  PulseType=Time based  Period=10  PulseWidth=0.1  PhaseDelay=2
  Switch : Switch  Criteria=u2 > Threshold
  Output : Outport
  wires:
  Switch/1 -> Output/1
  Constant/1 -> Switch/3
  Input/1 -> Switch/1
  Pulse Generator/1 -> Switch/2

== system v2021_10_27_Gear/Forze normali all'atterraggio/Subsystem5/logica reset1 ==
  note: se negli ultimi 6 timestep la distanza pista-ruota è negativa, smetti di resettare l'integratore
  note: Questa costante rappresenta un piccolo
      | margine alla posizione della ruota per la
      | procedura di reset logico.
  h : Inport
  Constant : Constant  Value=0
  Constant1 : Constant  Value=0.05
  Memory{,1..5} (6 alike) : Memory
  Sign{,1..5} (6 alike) : Signum
  Sum : Sum  Inputs=++++++
  Sum1 : Sum  Inputs=-+
  Sum2 : Sum  Inputs=|+-
  Switch : Switch  Threshold=-1
  segnale reset : Outport
  wires:
  Sum2/1 -> Memory/1, Sum1/2
  h/1 -> Sum2/1
  Constant1/1 -> Sum2/2
  Sum1/1 -> Switch/1
  Constant/1 -> Switch/3
  Switch/1 -> segnale reset/1
  Sum/1 -> Switch/2
  Sign5/1 -> Sum/6
  Sign4/1 -> Sum/5
  Sign3/1 -> Sum/4
  Sign2/1 -> Sum/3
  Sign1/1 -> Sum/2
  Sign/1 -> Sum/1
  Memory5/1 -> Sign5/1
  Memory4/1 -> Sign4/1, Memory5/1
  Memory3/1 -> Sign3/1, Memory4/1
  Memory2/1 -> Sign2/1, Memory3/1
  Memory1/1 -> Sign1/1, Memory2/1
  Memory/1 -> Sum1/1, Memory1/1, Sign/1

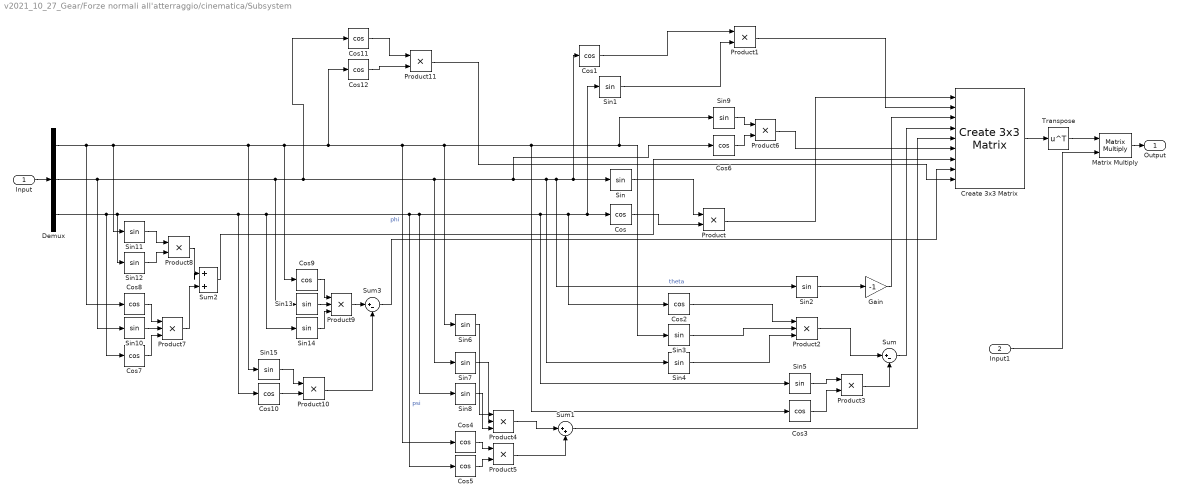
== system v2021_10_27_Gear/Forze normali all'atterraggio/cinematica/Subsystem ==
  Input : Inport
  Input1 : Inport  Port=2
  Cos{,1..12} (13 alike) : Trigonometry  Operator=cos
  Create 3x3 Matrix : sharedutil/Create 3x3 Matrix  aMode=aMode
  Demux : Demux  Outputs=3
  Gain : Gain  Gain=-1
  Matrix Multiply : Product  Multiplication=Matrix(*)
  Product{,1,3,5..6,8,10..11} (8 alike) : Product
  Product{2,4,7,9} (4 alike) : Product  Inputs=3
  Sin{,1..15} (16 alike) : Trigonometry
  Sum : Sum  Inputs=|+-
  Sum1 : Sum  Inputs=|++
  Sum2 : Sum  Inputs=|++
  Sum3 : Sum  Inputs=|+-
  Transpose : Math  Operator=transpose  SignedPower=on  SaturateOnIntegerOverflow=on
  Output : Outport  VectorParamsAs1DForOutWhenUnconnected=off
  wires:
  Transpose/1 -> Matrix Multiply/1
  Matrix Multiply/1 -> Output/1
  Input1/1 -> Matrix Multiply/2
  Create 3x3 Matrix/1 -> Transpose/1
  Product11/1 -> Create 3x3 Matrix/9
  Cos12/1 -> Product11/2
  Cos11/1 -> Product11/1
  Sum3/1 -> Create 3x3 Matrix/8
  Product10/1 -> Sum3/2
  Cos10/1 -> Product10/2
  Sin15/1 -> Product10/1
  Product9/1 -> Sum3/1
  Sin14/1 -> Product9/3
  Sin13/1 -> Product9/2
  Cos9/1 -> Product9/1
  Sum2/1 -> Create 3x3 Matrix/7
  Product8/1 -> Sum2/1
  Product7/1 -> Sum2/2
  Sin12/1 -> Product8/2
  Sin11/1 -> Product8/1
  Cos7/1 -> Product7/3
  Sin10/1 -> Product7/2
  Cos8/1 -> Product7/1
  Product6/1 -> Create 3x3 Matrix/6
  Cos6/1 -> Product6/2
  Sin9/1 -> Product6/1
  Sum1/1 -> Create 3x3 Matrix/5
  Product5/1 -> Sum1/2
  Product4/1 -> Sum1/1
  Cos5/1 -> Product5/2
  Cos4/1 -> Product5/1
  Sin8/1 -> Product4/3
  Sin7/1 -> Product4/2
  Sin6/1 -> Product4/1
  Sum/1 -> Create 3x3 Matrix/4
  Product3/1 -> Sum/2
  Cos3/1 -> Product3/2
  Sin5/1 -> Product3/1
  Sin4/1 -> Product2/3
  Cos2/1 -> Product2/1
  Product2/1 -> Sum/1
  Sin3/1 -> Product2/2
  Gain/1 -> Create 3x3 Matrix/3
  Demux/2 -> Sin/1, Cos1/1, Sin2/1, Sin4/1, Cos6/1, Sin7/1, Cos11/1, Sin13/1, Sin10/1  "theta"
  Sin2/1 -> Gain/1
  Product1/1 -> Create 3x3 Matrix/2
  Sin1/1 -> Product1/2
  Cos1/1 -> Product1/1
  Product/1 -> Create 3x3 Matrix/1
  Cos/1 -> Product/2
  Sin/1 -> Product/1
  Demux/3 -> Cos/1, Sin1/1, Cos2/1, Sin5/1, Sin8/1, Cos5/1, Sin14/1, Cos10/1, Sin12/1, Cos7/1  "psi"
  Demux/1 -> Sin11/1, Sin3/1, Sin9/1, Cos3/1, Sin6/1, Cos4/1, Cos12/1, Cos9/1, Sin15/1, Cos8/1  "phi"
  Input/1 -> Demux/1

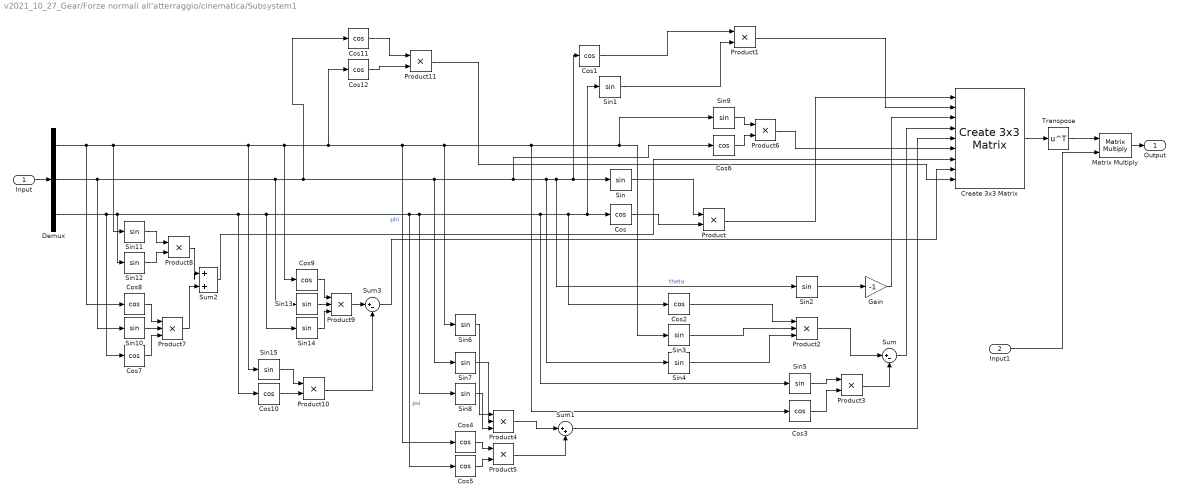
== system v2021_10_27_Gear/Forze normali all'atterraggio/cinematica/Subsystem1 ==
  Input : Inport
  Input1 : Inport  Port=2
  Cos{,1..12} (13 alike) : Trigonometry  Operator=cos
  Create 3x3 Matrix : sharedutil/Create 3x3 Matrix  aMode=aMode
  Demux : Demux  Outputs=3
  Gain : Gain  Gain=-1
  Matrix Multiply : Product  Multiplication=Matrix(*)
  Product{,1,3,5..6,8,10..11} (8 alike) : Product
  Product{2,4,7,9} (4 alike) : Product  Inputs=3
  Sin{,1..15} (16 alike) : Trigonometry
  Sum : Sum  Inputs=|+-
  Sum1 : Sum  Inputs=|++
  Sum2 : Sum  Inputs=|++
  Sum3 : Sum  Inputs=|+-
  Transpose : Math  Operator=transpose  SignedPower=on  SaturateOnIntegerOverflow=on
  Output : Outport  VectorParamsAs1DForOutWhenUnconnected=off
  wires:
  Transpose/1 -> Matrix Multiply/1
  Matrix Multiply/1 -> Output/1
  Input1/1 -> Matrix Multiply/2
  Create 3x3 Matrix/1 -> Transpose/1
  Product11/1 -> Create 3x3 Matrix/9
  Cos12/1 -> Product11/2
  Cos11/1 -> Product11/1
  Sum3/1 -> Create 3x3 Matrix/8
  Product10/1 -> Sum3/2
  Cos10/1 -> Product10/2
  Sin15/1 -> Product10/1
  Product9/1 -> Sum3/1
  Sin14/1 -> Product9/3
  Sin13/1 -> Product9/2
  Cos9/1 -> Product9/1
  Sum2/1 -> Create 3x3 Matrix/7
  Product8/1 -> Sum2/1
  Product7/1 -> Sum2/2
  Sin12/1 -> Product8/2
  Sin11/1 -> Product8/1
  Cos7/1 -> Product7/3
  Sin10/1 -> Product7/2
  Cos8/1 -> Product7/1
  Product6/1 -> Create 3x3 Matrix/6
  Cos6/1 -> Product6/2
  Sin9/1 -> Product6/1
  Sum1/1 -> Create 3x3 Matrix/5
  Product5/1 -> Sum1/2
  Product4/1 -> Sum1/1
  Cos5/1 -> Product5/2
  Cos4/1 -> Product5/1
  Sin8/1 -> Product4/3
  Sin7/1 -> Product4/2
  Sin6/1 -> Product4/1
  Sum/1 -> Create 3x3 Matrix/4
  Product3/1 -> Sum/2
  Cos3/1 -> Product3/2
  Sin5/1 -> Product3/1
  Sin4/1 -> Product2/3
  Cos2/1 -> Product2/1
  Product2/1 -> Sum/1
  Sin3/1 -> Product2/2
  Gain/1 -> Create 3x3 Matrix/3
  Demux/2 -> Sin/1, Cos1/1, Sin2/1, Sin4/1, Cos6/1, Sin7/1, Cos11/1, Sin13/1, Sin10/1  "theta"
  Sin2/1 -> Gain/1
  Product1/1 -> Create 3x3 Matrix/2
  Sin1/1 -> Product1/2
  Cos1/1 -> Product1/1
  Product/1 -> Create 3x3 Matrix/1
  Cos/1 -> Product/2
  Sin/1 -> Product/1
  Demux/3 -> Cos/1, Sin1/1, Cos2/1, Sin5/1, Sin8/1, Cos5/1, Sin14/1, Cos10/1, Sin12/1, Cos7/1  "psi"
  Demux/1 -> Sin11/1, Sin3/1, Sin9/1, Cos3/1, Sin6/1, Cos4/1, Cos12/1, Cos9/1, Sin15/1, Cos8/1  "phi"
  Input/1 -> Demux/1
